simulink library "rfports1"  (Simulink 6.0)
settings: Solver=ode45  SolverMode=SingleTasking  StartTime=0.0  StopTime=10.0  RelTol=1e-3
undefined symbols (not defined in the file or in its folder): models
libraries: rfprivate1 x11
settings Model: RequirementInfo=9  CovMetricSettings=d  Creator=tdelve  LastModifiedBy=fwei  ExtModeAutoUpdateStatusClock=off  ProdHWDeviceType=Specified
settings DataIOCC: SignalLoggingName=logsOut
settings OptimizationCC: BooleanDataType=off
settings DebuggingCC: CheckExecutionContextPreStartOutputMsg=on  CheckExecutionContextRuntimeOutputMsg=on  SolverPrmCheckMsg=none
settings HardwareCC: ProdHWDeviceType=Specified  TargetUnknown=on
settings ModelReferenceCC: UpdateModelReferenceTargets=IfOutOfDate
settings SFSimCC: SFSimApplyToAllLibs=on  SFSimBuildMode=Incremental

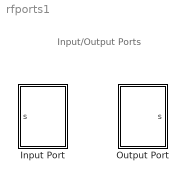
== system rfports1 ==
  note: Input/Output Ports
  Input Port : Subsystem  Description=source block  PropExecContextAcrossSSBoundary=on  mask(Input Port){MaxLength=128, Fc=2e9, Ts=1e-7, Zs=50, NoiseFlag=off, seed=67987, GoToTag=RFTag}
      mask prompts: MaxLength "Max length of impulse response:"; Fc "Center frequency (Hz):"; Ts "Sample time (s):"; Zs "Source impedance:"; NoiseFlag "Add noise"; seed "Initial seed:"; GoToTag "Tag:"
      mask help:
      | Connection block from Simulink to RF Blockset physical blocks.
      |
      | The first three parameters determine the frequency range of interest.
      mask init:
      | set_param([gcb '/Goto'],'GoToTag',GoToTag); 
      | mStr = rfblksanalyze1(gcb,'rfInitInput');
      | if(~isempty(mStr.emsg)) error(mStr.emsg); end
      | if(~isempty(mStr.wmsg)) warning(mStr.wmsg); end
      settings: DeleteFcn=rfblksanalyze1(gcb,'rfDeleteInput');
      mask Help: helpview(rfbhelp)
      mask CallbackString: ||||rfblksanalyze1(gcb,'rfNoiseOn');||
      mask Display: disp('Input\nPort');
  Output Port : Subsystem  PropExecContextAcrossSSBoundary=on  mask(Output Port){Zl=50, num_Models=0, GoToTag=RFTag, DisplayData=off, PlotFreq=Derived from Input Port parameters, Freq=1e9:1e8:3e9, AllPlotType=Composite data, NoBudgetPlot=Composite data, NetworkData=S11, SmithData=S11, PolarData=S11, ComplexFormat=Magnitude (decibels), DBFormat=Magnitude (decibels), DBMFormat=dBm, NoneFormat=None}
      mask prompts: Zl "Load impedance:"; num_Models "Number of models:"; GoToTag "Tag:"; DisplayData "Plot the network parameters of the RF system"; PlotFreq "Source of frequency data:"; Freq "Frequency data (Hz):"; AllPlotType "Plot type:"; NoBudgetPlot "Plot type:"; NetworkData "Parameter:"; SmithData "Parameter:"; PolarData "Parameter:"; ComplexFormat "Format:"; DBFormat "Format:"; DBMFormat "Format:"; NoneFormat "Format:"
      mask help:
      | Connection block from RF Blockset physical blocks to Simulink.
      |
      | After running a simulation, various parameters of the RF system that is delimited by an Input Port block and this Output Port block can be visualized.
      mask init:
      | set_param([gcb '/From'],'GotoTag',GoToTag); 
      | [mStr, models, rfsys] = rfblksanalyze1(gcb,'rfInitOutput');
      | if(~isempty(mStr.emsg)) error(mStr.emsg); end
      | if(~isempty(mStr.wmsg)) warning(mStr.wmsg); end
      settings: DeleteFcn=rfblksanalyze1(gcb,'rfDeleteOutput');
      mask Help: helpview(rfbhelp)
      mask StyleString: edit,edit,edit,checkbox,popup(Derived from Input Port parameters|User specified),edit,popup(Composite data|X-Y plane|Polar plane|Z Smith chart|Y Smith chart|ZY Smith chart),popup(Composite data|X-Y plane|Polar plane|Z Smith chart|Y Smith chart|ZY Smith chart),popup(S11|S12|S21|S22|VSWRIn|VSWROut|OIP3|NF),popup(S11|S22),popup(S11|S12|S21|S22),popup(Magnitude (decibels)|Magnitude (linear)|Angle (degrees)|Real|Imaginary),popup(Magnitude (decibels)|None),popup(dBm|W|mW),popup(None)
      mask CallbackString: |||rfblksanalyze1(gcb,'rfUpdateBlockMask');|rfblksanalyze1(gcb,'rfUpdateBlockMask');||rfblksanalyze1(gcb,'rfUpdateBlockMask');|rfblksanalyze1(gcb,'rfUpdateBlockMask');|rfblksanalyze1(gcb,'rfUpdateBlockMask');|rfblksanalyze1(gcb,'rfUpdateBlockMask');|rfblksanalyze1(gcb,'rfUpdateBlockMask');||||
      mask Display: disp('Output\nPort');

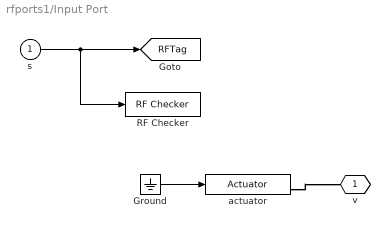
== system rfports1/Input Port ==
  s : Inport  LatchInput=off
  Ground : Ground
  RF Checker : rfprivate1/RF Checker  ts=Ts
  actuator : Actuator  PhysicalDomain=rfsystemsdomain  SubClassName=source  PortType=p1
  v : PMIOPort  Orientation=left  Port=1  Side=Right
  tag scope: RFTag=global
  wires:
  s/1 -> [RFTag], RF Checker/1
  Ground/1 -> actuator/1
  connections:
  actuator/RConn1 -- v/RConn1

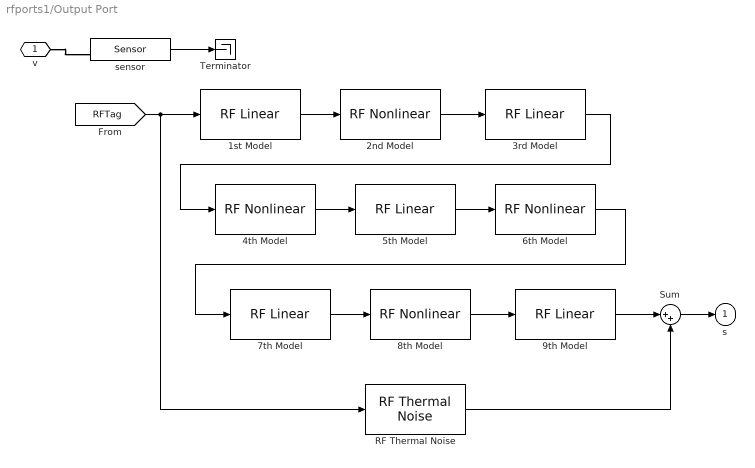
== system rfports1/Output Port ==
  1st Model : rfprivate1/RF Linear  model=models{1}
  2nd Model : rfprivate1/RF Nonlinear  model=models{2}
  3rd Model : rfprivate1/RF Linear  model=models{3}
  4th Model : rfprivate1/RF Nonlinear  model=models{4}
  5th Model : rfprivate1/RF Linear  model=models{5}
  6th Model : rfprivate1/RF Nonlinear  model=models{6}
  7th Model : rfprivate1/RF Linear  model=models{7}
  8th Model : rfprivate1/RF Nonlinear  model=models{8}
  9th Model : rfprivate1/RF Linear  model=models{9}
  RF Thermal Noise : rfprivate1/RF Thermal Noise  model=rfsys
  Sum : Sum  Inputs=|++
  Terminator : Terminator
  sensor : Sensor  PhysicalDomain=rfsystemsdomain  SubClassName=sink  PortType=p1
  v : PMIOPort  Port=1  Side=Left
  s : Outport  InitialOutput=0
  wires:
  RF Thermal Noise/1 -> Sum/2
  9th Model/1 -> Sum/1
  Sum/1 -> s/1
  6th Model/1 -> 7th Model/1
  5th Model/1 -> 6th Model/1
  3rd Model/1 -> 4th Model/1
  7th Model/1 -> 8th Model/1
  8th Model/1 -> 9th Model/1
  4th Model/1 -> 5th Model/1
  1st Model/1 -> 2nd Model/1
  2nd Model/1 -> 3rd Model/1
  [RFTag] -> RF Thermal Noise/1, 1st Model/1
  sensor/1 -> Terminator/1
  connections:
  v/RConn1 -- sensor/LConn1
